simulink model "power_arrester"  (Simulink 6.0)
settings: Solver=ode23tb  SolverMode=SingleTasking  StartTime=0.0  StopTime=.2  FixedStep=40e-6  RelTol=1e-4
libraries: powerlib x15, simulink x1
settings Model: Creator=patrice  LastModifiedBy=batserve  ExtModeTrigMode=oneshot  ExtModeArmWhenConnect=off  ExtModeAutoUpdateStatusClock=off
settings DataIOCC: LimitDataPoints=off  SignalLoggingName=sigsOut  OutputTimes=0.00001
settings OptimizationCC: BooleanDataType=off
settings DebuggingCC: AlgebraicLoopMsg=none  SolverPrmCheckMsg=none
settings HardwareCC: TargetUnknown=on
settings RTWCC: TemplateMakefile=grt_unix.tmf

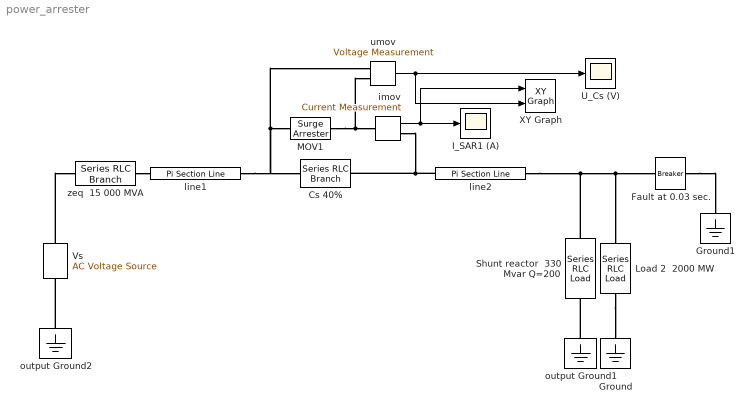
== system power_arrester ==
  " MOV1" : powerlib/Elements/Surge Arrester  ProtectionVoltage=185e3  Columns=30  ReferenceCurrent=500  Segment1=[.955 50]  Segment2=[1.0 25]  Segment3=[.9915 16.5]  Measurements=None  MoreParameters=off  BreakLoop=off
      settings: AttributesFormatString=\n
  Cs 40% : powerlib/Elements/Series RLC Branch  PhysicalDomain=powersysdomain  SubClassName=unknown  LeftPortType=p1  RightPortType=p1  LConnTagsString=__new0  RConnTagsString=__new0  Resistance=0  Inductance=0  Capacitance=101.4e-6  Measurements=None
  Fault at 0.03 sec. : powerlib/Elements/Breaker  BreakerResistance=1  InitialState=0  SnubberResistance=inf  SnubberCapacitance=0  SwitchingTimes="[ 30e-3  100e-3 ]"  External=off  Measurements=None
      settings: AttributesFormatString=\n
  Ground : powerlib/Elements/Ground  Orientation=down  PhysicalDomain=powersysdomain  SubClassName=unknown  LeftPortType=p1  RightPortType=p1  LConnTagsString=a
  Ground1 : powerlib/Elements/Ground  Orientation=down  PhysicalDomain=powersysdomain  SubClassName=unknown  LeftPortType=p1  RightPortType=p1  LConnTagsString=a
  I_SAR1 (A) : Scope
      settings: TickLabels=on  TimeRange=0.1  YMin=-5000  YMax=10000  DataFormat=Array  MaxDataPoints=500000
  Load 2  2000 MW : powerlib/Elements/Series RLC Load  Orientation=down  PhysicalDomain=powersysdomain  SubClassName=unknown  LeftPortType=p1  RightPortType=p1  LConnTagsString=a  RConnTagsString=__new0  NominalVoltage=735e3/sqrt(3)  NominalFrequency=60  ActivePower=2000e6/3  InductivePower=0  CapacitivePower=0  Measurements=None
  Shunt reactor  330 Mvar Q=200 : powerlib/Elements/Series RLC Load  Orientation=up  PhysicalDomain=powersysdomain  SubClassName=unknown  LeftPortType=p1  RightPortType=p1  LConnTagsString=a  RConnTagsString=__new0  NominalVoltage=735e3/sqrt(3)  NominalFrequency=60  ActivePower=330e6/3/200  InductivePower=330e6/3  CapacitivePower=0  Measurements=None
  U_Cs (V) : Scope
      settings: TickLabels=on  TimeRange=0.1  YMin=-200000  YMax=200000  DataFormat=Array  MaxDataPoints=500000
  Vs : powerlib/Electrical Sources/AC Voltage Source  Description=source block  Orientation=up  Amplitude=735e3/sqrt(3)*sqrt(2)  Phase=0  Frequency=60  SampleTime=0  Measurements=None
      settings: AttributesFormatString=\n
  XY Graph : simulink/Sinks/XY Graph  xmin=-6000  xmax=6000  ymin=-2e5  ymax=2e5  st=-1
  imov : powerlib/Measurements/Current Measurement  Tag=PoWeRsYsTeMmEaSuReMeNt  PhasorSimulation=off  OutputType=Magnitude  PSBequivalent=0
  line1 : powerlib/Elements/Pi Section Line  PhysicalDomain=powersysdomain  SubClassName=unknown  LeftPortType=p1  RightPortType=p1  LConnTagsString=__new0  RConnTagsString=__new0  Frequency=60  Resistance=0.011  Inductance=0.8674e-3  Capacitance=13.41e-9  Length=100  PiSections=2  Measurements=None
      settings: AttributesFormatString=\n
  line2 : powerlib/Elements/Pi Section Line  PhysicalDomain=powersysdomain  SubClassName=unknown  LeftPortType=p1  RightPortType=p1  LConnTagsString=__new0  RConnTagsString=__new0  Frequency=60  Resistance=0.011  Inductance=0.8674e-3  Capacitance=13.41e-9  Length=100  PiSections=2  Measurements=None
      settings: AttributesFormatString=\n
  output Ground1 : powerlib/Elements/Ground  Orientation=down  PhysicalDomain=powersysdomain  SubClassName=unknown  LeftPortType=p1  RightPortType=p1  LConnTagsString=a
  output Ground2 : powerlib/Elements/Ground  Orientation=down  PhysicalDomain=powersysdomain  SubClassName=unknown  LeftPortType=p1  RightPortType=p1  LConnTagsString=a
  umov : powerlib/Measurements/Voltage Measurement  Tag=PoWeRsYsTeMmEaSuReMeNt  PhasorSimulation=off  OutputType=Magnitude  PSBequivalent=0
  zeq  15 000 MVA : powerlib/Elements/Series RLC Branch  PhysicalDomain=powersysdomain  SubClassName=unknown  LeftPortType=p1  RightPortType=p1  LConnTagsString=__new0  RConnTagsString=__new0  Resistance=3.6  Inductance=95.5e-3  Capacitance=inf  Measurements=None
  wires:
  umov/1 -> U_Cs (V)/1, XY Graph/2
  imov/1 -> I_SAR1 (A)/1, XY Graph/1
  connections:
  Vs/RConn1 -- zeq  15 000 MVA/LConn1
  output Ground2/LConn1 -- Vs/LConn1
  zeq  15 000 MVA/RConn1 -- line1/LConn1
  output Ground1/LConn1 -- Shunt reactor  330 Mvar Q=200/LConn1
  line2/RConn1 -- Fault at 0.03 sec./LConn1 -- Load 2  2000 MW/LConn1 -- Shunt reactor  330 Mvar Q=200/RConn1
  Load 2  2000 MW/RConn1 -- Ground/LConn1
  Fault at 0.03 sec./RConn1 -- Ground1/LConn1
  line2/LConn1 -- Cs 40%/RConn1 -- imov/RConn1
  line1/RConn1 -- Cs 40%/LConn1 -- " MOV1"/LConn1 -- umov/LConn1
  " MOV1"/RConn1 -- imov/LConn1 -- umov/LConn2
